simulink model "QD2_IOCheck_AM32ESC_R2022b"  (R2022b)
settings: Solver=ode2  StartTime=0.0  StopTime=inf  FixedStep=1/1000  RelTol=1e-3  EnableMultiTasking=on
undefined symbols (not defined in the file): datetime, HIL, log_QD2_, m, qc_get_step_size, saved_data
libraries: quarc_library x71, simulink x11, simulink_extras x9
(part 2 of 3)

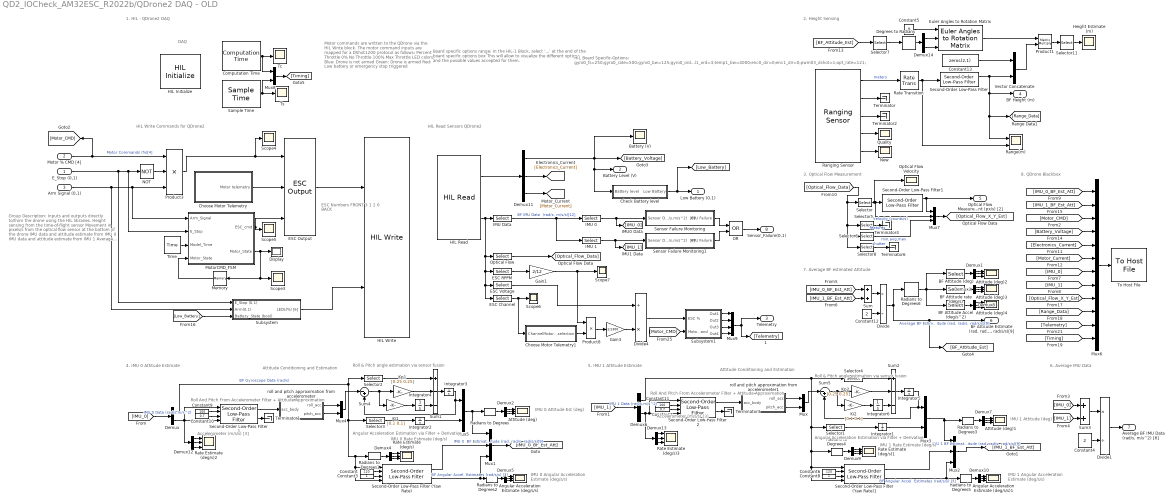
== system QD2_IOCheck_AM32ESC_R2022b/QDrone2 DAQ - OLD ==
  note: 1. HIL - QDrone2 DAQ
  note: HIL Write Commands for QDrone2
  note: ESC Numbers
      |
      | FRONT
      | 3 1
      |
      | 2 0
      | BACK
  note: DAQ
  note: HIL Read Sensors QDrone2
  note: 2. Height Sensing
  note: 3. Optical Flow Measurement
  note: Angular Acceleration Estimation via Filter + Derivative
  note: Roll And Pitch From Accelerometer Filter + Attitude Approximation
  note: Attitude Conditioning and Estimation
  note: 5. IMU 1 Attitude Estimate
  note: IMU 0
      | Rate Estimate (deg/s)
  note: 7. Average BF estimated Attitude
  note: Accelerometer (m/s/s) [3]
  note: Accelerometer (m/s/s) [3]
  note: Roll & Pitch angle estimation via sensor fusion
  note: IMU 1
      | Angular Acceleration
      | Estimate (deg/s/s)
  note: Roll And Pitch From Accelerometer Filter + Attitude Approximation
  note: IMU 1
      | Attitude (deg)
  note: IMU 0
      | Angular Acceleration
      | Estimate (deg/s/s)
  note: Roll & Pitch angle estimation via sensor fusion
  note: Attitude Conditioning and Estimation
  note: 4. IMU 0 Attitude Estimate
  note: IMU 0
      | Attitude Est (deg)
  note: 8. QDrone Blackbox
  note: Angular Acceleration Estimation via Filter + Derivative
  note: 6. Average IMU Data
  note: IMU 1
      | Rate Estimate (deg/s)
  note: Motor commands are written to the QDrone via the HIL Write block. The motor command inputs are mapped for a DShot1200 protocol as follows:
      |
      | Percent Throttle
      | 0% No Throttle
      | 100% Max Throttle
      |
      | LED colors:
      | Blue: Drone is not armed
      | Green: Drone is armed
      | Red: Low battery or emergency stop triggered
  note: Board specific options range:
      |
      | In the HIL-1 Block,
      | select '...' at the end of the board specific options box
      | This will allow to visualize the different options
      | and the possible values accepted for them.
  note: HIL Board Specific-Options:
      | gyro0_fs=250;gyro0_rate=500;gyro0_bw=125;gyro0_ord=3;accel0_fs=16;accel0_rate=1000;accel0_bw=400;accel0_ord=3;temp0_bw=4000;gyro1_fs=250;gyro1_rate=500;gyro1_bw=125;gyro1_ord=3;accel1_fs=16;accel1_rate=1000;accel1_bw=400;accel1_ord=3;temp1_bw=4000;enc0_dir=0;enc1_dir=0;pwm03_dshot=1;opt_rate=121;
  note: Group Description:
      |
      | Inputs and outputs directly to/from the drone using the HIL libraries.
      | Height sensing from the time-of-flight sensor
      | Movement in pixels/s from the optical flow sensor at the bottom of the drone
      | IMU data and attitude estimate from IMU 0
      | IMU data and attitude estimate from IMU 1
      | Average of both IMU outputs
      | Average body frame attitude from IMU data
      | Blackbox saving all relevant values
  E_Stop (0,1) : Inport
  Motor % CMD [4] : Inport  Port=2
  Arm Signal (0,1) : Inport  Port=3
  Angular Acceleration Estimate (deg/s/s) : Scope  NumInputPorts=3
  Angular Acceleration Estimate (deg/s/s)1 : Scope  NumInputPorts=3
  Attitude (deg){,1..4} (5 alike) : Scope  NumInputPorts=3
  BF Attitude (deg) : Selector  InputPortWidth=9  IndexOptions=Index vector (dialog)  Indices=[1:3]  OutputSizes=1
  BF Attitude Accel (deg/s^2) : Selector  InputPortWidth=9  IndexOptions=Index vector (dialog)  Indices=[7:9]  OutputSizes=1
  BF Attitude rate (deg/s) : Selector  InputPortWidth=9  IndexOptions=Index vector (dialog)  Indices=[4:6]  OutputSizes=1
  Battery (V) : Scope
  Check Battery level : Subsystem
  Choose Motor Telemetry : Subsystem
  Choose Motor Telemetry1 : Subsystem
  Computation Time : quarc_library/Sources/Time/Computation Time  sample_time=qc_get_step_size  use_model=on  use_cpu_time=off
  Constant : Constant  Value=120
  Constant10 : Constant  Value=0.7
  Constant11 : Constant  Value=100
  Constant12 : Constant  Value=2
  Constant13 : Constant  Value=zeros(2,1)
  Constant3 : Constant
  Constant4 : Constant  Value=2
  Constant5 : Constant  Value=0
  Constant6 : Constant  Value=120
  Constant7 : Constant  Value=0.7
  Constant8 : Constant
  Constant9 : Constant  Value=100
  Degrees to Radians : simulink_extras/Transformations/Degrees to Radians
  Demux : Demux  Outputs=[3,3]
  Demux{1..5,7..13} (12 alike) : Demux  Outputs=3
  Demux14 : Demux  Outputs=2
  Demux6 : Demux  Outputs=[3,3]
  Display : Display
  Divide : Product  Inputs=*/
  Divide1 : Product  Inputs=*/
  Divide4 : Product  Inputs=/*
  ESC Channel : Selector  InputPortWidth=22  IndexOptions=Index vector (dialog)  Indices=[22]  OutputSizes=1
  ESC Output : quarc_library/Data Acquisition/Generic/Transformations/ESC Output  protocol=DShot (raw)
      settings: AttributesFormatString=%<protocol>  SourceProductName=QUARC Targets
  ESC RPPM : Selector  InputPortWidth=22  IndexOptions=Index vector (dialog)  Indices=[20]  OutputSizes=1
  ESC Voltage : Selector  InputPortWidth=22  IndexOptions=Index vector (dialog)  Indices=[21]  OutputSizes=1
  Euler Angles to Rotation Matrix : quarc_library/Math Operations/Matrices/Euler Angles to Rotation Matrix  menu_order=Relative Z-X-Y
      settings: SourceProductName=QUARC Targets
  Gain1 : Gain  Gain=2/12
  Gain3 : Gain  Gain=1/1300
  HIL Initialize : quarc_library/Data Acquisition/Generic/Configuration/HIL Initialize  object_name=HIL-1  board_type=qdrone2  board_number=0  board_options=gyro0_fs=250;gyro0_rate=500;gyro0_bw=125;gyro0_ord=3;accel0_fs=16;accel0_rate=1000;accel0_bw=400;accel0_ord=3;temp0_bw=4000;gyro1_fs=250;gyro1_rate=500;gyro1_bw=125;gyro1_ord=3;accel1_fs=16;accel1_rate=1000;accel1_bw=400;accel1_ord=3;temp1_bw=4000;enc0_dir=0;enc1_dir=0;pwm03_dshot=1;opt_rate=121;  exclusive=off  active=on  hardware_clocks=[]  clock_modes=[]  initial_clock_frequencies=[]  set_clock_params_at_start=off  set_clock_params_at_switch_in=off  set_clock_frequencies_at_start=off  set_clock_frequencies_at_switch_in=off  analog_input_channels=[0:3]  analog_input_configurations=[]  analog_input_maximums=[3.3]  analog_input_minimums=[0]  set_analog_input_params_at_start=off  set_analog_input_params_at_switch_in=off  analog_output_channels=[]  analog_output_maximums=[]  analog_output_minimums=[]  initial_analog_outputs=[]  final_analog_outputs=[]  watchdog_analog_outputs=[]  set_analog_output_params_at_start=off  set_analog_output_params_at_switch_in=off  set_analog_outputs_at_start=off  set_analog_outputs_at_switch_in=off  set_analog_outputs_at_terminate=off  set_analog_outputs_at_switch_out=off  set_analog_outputs_on_watchdog=off  digital_input_channels=[0:5]  digital_output_channels=[6:11]  digital_output_configuration=[]  initial_digital_outputs=[0]  final_digital_outputs=[0]  watchdog_digital_outputs=[0 0 0 0 0 0]  set_digital_output_params_at_start=off  set_digital_output_params_at_switch_in=off  set_digital_outputs_at_start=on  set_digital_outputs_at_switch_in=off  set_digital_outputs_at_terminate=on  set_digital_outputs_at_switch_out=off  set_digital_outputs_on_watchdog=off  encoder_channels=[0:1]  quadrature=[4]  encoder_filter_frequency=100e6/1  initial_encoder_counts=[0]  set_encoder_params_at_start=on  set_encoder_params_at_switch_in=off  set_encoder_counts_at_start=on  set_encoder_counts_at_switch_in=off  pwm_channels=[0:5]  pwm_modes=[6 6 6 6 0 0]  pwm_frequency=1.2e6  pwm_configuration=[0]  pwm_alignment=[0]  pwm_polarity=[1]  pwm_leading_deadband=[]  pwm_trailing_deadband=[]  initial_pwm_outputs=[0]  final_pwm_outputs=[0]  watchdog_pwm_outputs=[0]  set_pwm_params_at_start=on  set_pwm_params_at_switch_in=off  set_pwm_outputs_at_start=on  set_pwm_outputs_at_switch_in=off  set_pwm_outputs_at_terminate=on  set_pwm_outputs_at_switch_out=off  set_pwm_outputs_on_watchdog=on  other_output_channels=[]  initial_other_outputs=[]  final_other_outputs=[]  watchdog_other_outputs=[]  set_other_outputs_at_start=on  set_other_outputs_at_switch_in=off  set_other_outputs_at_terminate=on  set_other_outputs_at_switch_out=off  set_other_outputs_on_watchdog=off
  HIL Read : quarc_library/Data Acquisition/Generic/Immediate I//O/HIL Read  object_name=HIL-1  analog_channels=[3 1:2]  encoder_channels=[]  digital_channels=[]  other_channels=[3000:3002 4000:4002 3003:3005 4003:4005 17000:17006 17008:17009 17007]  sample_time=qc_get_step_size  active=on  vector_output=on  data_type_mode=Inherit via back propagation  encoder_data_type=double  digital_data_type=boolean
  HIL Write : quarc_library/Data Acquisition/Generic/Immediate I//O/HIL Write  object_name=HIL-1  analog_channels=[]  pwm_channels=[0:3]  digital_channels=[6:11]  other_channels=[]  sample_time=-1  active=off  vector_input=on
  Height Estimate (m) : Scope
  IMU 0 : Selector  InputPortWidth=12  IndexOptions=Index vector (dialog)  Indices=[1:6]  OutputSizes=1
  IMU 1 : Selector  InputPortWidth=12  IndexOptions=Index vector (dialog)  Indices=[7:12]  OutputSizes=1
  IMU Data : Selector  InputPortWidth=22  IndexOptions=Index vector (dialog)  Indices=[1:12]  OutputSizes=1
  Integrator{1..6} (6 alike) : Integrator
  Ki1 : Gain  Gain=[0.1 0.1]
  Ki2 : Gain  Gain=[0.1 0.1]
  Kp1 : Gain  Gain=[0.25 0.25]
  Kp2 : Gain  Gain=[0.25 0.25]
  Memory : Memory
  MotorCMD_FSM : MATLAB Function  TreatAsAtomicUnit=on
  Mux{,3..5,8} (5 alike) : Mux  Inputs=2
  Mux1 : Mux  Inputs=3
  Mux2 : Mux  Inputs=3
  Mux6 : Mux  Inputs=12
  Mux7 : Mux  Inputs=3
  Mux9 : Mux
  NOT : Logic  Operator=NOT  IconShape=distinctive  AllPortsSameDT=off  OutDataTypeStr=boolean
  New : Scope
  OR : Logic  Operator=OR  AllPortsSameDT=off  OutDataTypeStr=boolean
  Optical Flow : Selector  InputPortWidth=22  IndexOptions=Index vector (dialog)  Indices=[13:19]  OutputSizes=1
  Optical Flow Velocity : Scope
  Product1 : Product  Multiplication=Matrix(*)
  Product3 : Product  Inputs=3
  Product8 : Product
  Quality : Scope
  Radians to Degrees{,1..6} (7 alike) : simulink_extras/Transformations/Radians to Degrees
  Range(m) : Scope  NumInputPorts=2
  Ranging Sensor : quarc_library/Devices/Third-Party/Sensors/Ranging Sensor  sensor_type=VL53L1X Time-of-flight  uri=i2c-cpu://localhost:0?address='0x29',baud='400000',memsize='512'  ranging_distance=Long  timing_budget=0.033  measurement_period=0.040  output_mode=Fixed-size output  samples_per_revolution=1300  max_distance=0.050  max_angle=5  sample_time=qc_get_step_size * ceil(1/121/ qc_get_step_size)  show_versions=off  active=on
      settings: SourceProductName=QUARC Targets
  Rate Estimate (deg/s){,1..3} (4 alike) : Scope  NumInputPorts=3
  Rate Transition : RateTransition
  Sample Time : quarc_library/Sources/Time/Sample Time  Priority=-99  sample_time=qc_get_step_size
  Scope{3..7} (5 alike) : Scope
  Second-Order Low-Pass Filter : quarc_library/Continuous/Second-Order Low-Pass Filter  params_source=Internal (dialog parameters)  input_width=100  input_zeta=0.7  input_init=0
  Second-Order Low-Pass Filter (Yaw Rate) : quarc_library/Continuous/Second-Order Low-Pass Filter  params_source=External (input ports)  input_width=200  input_zeta=1  input_init=0
  Second-Order Low-Pass Filter (Yaw Rate)1 : quarc_library/Continuous/Second-Order Low-Pass Filter  params_source=External (input ports)  input_width=200  input_zeta=1  input_init=0
  Second-Order Low-Pass Filter 1 : quarc_library/Continuous/Second-Order Low-Pass Filter  params_source=External (input ports)  input_width=50  input_zeta=1  input_init=0
  Second-Order Low-Pass Filter 2 : quarc_library/Continuous/Second-Order Low-Pass Filter  params_source=External (input ports)  input_width=50  input_zeta=1  input_init=0
  Second-Order Low-Pass Filter1 : quarc_library/Continuous/Second-Order Low-Pass Filter  params_source=Internal (dialog parameters)  input_width=45  input_zeta=1.5  input_init=0
  Selector : Selector  InputPortWidth=7  IndexOptions=Index vector (dialog)  Indices=[1 2]  OutputSizes=1
  Selector1 : Selector  InputPortWidth=3  IndexOptions=Index vector (dialog)  Indices=[3]  OutputSizes=1
  Selector11 : Selector  InputPortWidth=3  IndexOptions=Index vector (dialog)  Indices=[3]  OutputSizes=1
  Selector2 : Selector  InputPortWidth=3  IndexOptions=Index vector (dialog)  Indices=[1,2]  OutputSizes=1
  Selector3 : Selector  InputPortWidth=3  IndexOptions=Index vector (dialog)  Indices=[3]  OutputSizes=1
  Selector4 : Selector  InputPortWidth=3  IndexOptions=Index vector (dialog)  Indices=[1,2]  OutputSizes=1
  Selector5 : Selector  InputPortWidth=7  IndexOptions=Index vector (dialog)  Indices=[3]  OutputSizes=1
  Selector6 : Selector  InputPortWidth=7  IndexOptions=Index vector (dialog)  Indices=[4 5 6]  OutputSizes=1
  Selector7 : Selector  InputPortWidth=9  IndexOptions=Index vector (dialog)  Indices=[1,2]  OutputSizes=1
  Selector8 : Selector  InputPortWidth=7  IndexOptions=Index vector (dialog)  Indices=[7]  OutputSizes=1
  Sensor Failure Monitoring : Subsystem
  Sensor Failure Monitoring1 : Subsystem
  Subsystem : Subsystem
  Subsystem1 : Subsystem
  Sum : Sum
  Sum1 : Sum  Inputs=+--
  Sum2 : Sum  Inputs=+--
  Sum3 : Sum
  Sum4 : Sum  Inputs=|-+
  Sum5 : Sum  Inputs=|-+
  Tc : Scope
  Terminator{,1..4,6} (6 alike) : Terminator
  Time : quarc_library/Sources/Time/Time  time_source=Wall clock  sample_time=qc_get_step_size
  To Host File : quarc_library/Sinks/To Host/To Host File  file_name=saved_data/%m/QDrone2_%{date}_%{time}.mat  variable_name=QDrone_data  decimation=1  sample_time=-1  file_format=MAT-file v.4  options=No header or footer  append=off  final_file_name=saved_data/QDrone2_IO_Check_2021b/QDrone2_10-Apr-2023_14-56-11.mat  bitrate=2000000
  Ts : Scope
  Vector Concatenate : Concatenate
  roll and pitch approximation from accelerometer : MATLAB Function  TreatAsAtomicUnit=on
  roll and pitch approximation from accelerometer1 : MATLAB Function  TreatAsAtomicUnit=on
  Low Battery (0,1) : Outport
  Battery Level (V) : Outport  Port=2
  Telemetry : Outport  Port=3
  "BF Height (m) " : Outport  Port=4
  Optical Flow Measurement (px/s) [2] : Outport  Port=5
  "BF Attitude Estimate (rad, rad/s, rad/s/s)[9]" : Outport  Port=6
  "Average BF IMU Data (rad/s, m/s^2) [6]" : Outport  Port=7
  Sensor_Failure(0,1) : Outport  Port=8
  wires:
  Subsystem/1(LEDs(%) [6]) -> HIL Write/2
  [Low_Battery] -> Subsystem/3(Battery_State (bool))
  Arm Signal (0,1)/1 -> Product3/3, MotorCMD_FSM/1(Arm_Signal), Subsystem/2("Arm(0,1) ")
  NOT/1 -> Product3/2
  Motor % CMD [4]/1 -> [Motor_CMD], Product3/1  "Motor Commands (%)[4]"
  E_Stop (0,1)/1 -> Subsystem/1(E_Stop (0,1)), MotorCMD_FSM/2(E_Stop), NOT/1
  Time/1 -> MotorCMD_FSM/3(Model_Time)
  MotorCMD_FSM/2(Motor_State) -> Scope3/1, Memory/1, Display/1
  Memory/1 -> MotorCMD_FSM/4("Motor_State ")
  Choose Motor Telemetry/1(Motor telemetry) -> ESC Output/2
  ESC Output/1 -> HIL Write/1
  MotorCMD_FSM/1(ESC_cmd) -> ESC Output/3, Scope5/1
  Product3/1 -> Scope4/1, ESC Output/1
  OR/1 -> Sensor_Failure(0,1)/1
  Gain3/1 -> Divide4/2
  [Motor_CMD] -> Subsystem1/2(Motor command)
  ESC Channel/1 -> Scope6/1, Choose Motor Telemetry1/1(Channel)
  HIL Read/2 -> IMU Data/1, ESC RPPM/1, ESC Voltage/1, ESC Channel/1, Optical Flow/1
  ESC RPPM/1 -> Gain1/1
  Gain1/1 -> Product8/1, Scope7/1
  Product8/1 -> Gain3/1
  ESC Voltage/1 -> Divide4/1
  Choose Motor Telemetry1/1(Motor selection) -> Product8/2
  Divide4/1 -> Subsystem1/1(ESC %)
  Check Battery level/1(Low Battery) -> [Low_Battery], Low Battery (0,1)/1
  IMU 1/1 -> [IMU_1], Sensor Failure Monitoring1/1(Sensor Data (rad/s,m/s^2)  [6])
  Sensor Failure Monitoring/1(IMU Failure) -> OR/1
  IMU 0/1 -> [IMU_0], Sensor Failure Monitoring/1(Sensor Data (rad/s,m/s^2)  [6])
  Demux11/1 -> Battery Level (V)/1, Check Battery level/1(Battery level), [Battery_Voltage], Battery (V)/1
  HIL Read/1 -> Demux11/1
  Demux11/3 -> [Motor_Current]
  Demux11/2 -> [Electronics_Current]
  Mux9/1 -> Telemetry/1, [Telemetry]
  Sensor Failure Monitoring1/1(IMU Failure) -> OR/2
  Subsystem1/4(Out4) -> Mux9/4
  IMU Data/1 -> IMU 1/1, IMU 0/1  "BF IMU Data  (rad/s, m/s/s)[12]"
  Subsystem1/2(Out2) -> Mux9/2
  Subsystem1/1(Out1) -> Mux9/1
  Subsystem1/3(Out3) -> Mux9/3
  Optical Flow/1 -> [Optical_Flow_Data]
  Ranging Sensor/2 -> Terminator/1
  Rate Transition/1 -> Range(m)/2, Second-Order Low-Pass Filter/1
  Constant5/1 -> Euler Angles to Rotation Matrix/1
  Selector7/1 -> Degrees to Radians/1
  Euler Angles to Rotation Matrix/1 -> Product1/1
  Ranging Sensor/3 -> Terminator2/1
  Second-Order Low-Pass Filter1/1 -> Optical Flow Measurement (px/s) [2]/1, Mux7/1
  Vector Concatenate/1 -> Product1/2
  Second-Order Low-Pass Filter/1 -> [Range_Data], Range(m)/1, "BF Height (m) "/1, Vector Concatenate/2
  Ranging Sensor/4 -> Quality/1
  Ranging Sensor/1 -> Rate Transition/1  "meters"
  Demux14/2 -> Euler Angles to Rotation Matrix/3
  Product1/1 -> Selector11/1
  Degrees to Radians/1 -> Demux14/1
  Selector11/1 -> Height Estimate (m)/1
  [Optical_Flow_Data] -> Selector/1, Selector8/1, Selector6/1, Selector5/1
  Ranging Sensor/5 -> New/1
  Demux14/1 -> Euler Angles to Rotation Matrix/2
  Constant13/1 -> Vector Concatenate/1
  [BF_Attitude_Est] -> Selector7/1
  BF Attitude rate (deg/s)/1 -> Demux3/1
  Demux12/3 -> Rate Estimate (deg/s)2/3
  Radians to Degrees2/1 -> Demux5/1
  Demux1/1 -> Attitude (deg)2/1
  [IMU_0] -> Sum3/1
  Demux12/1 -> Rate Estimate (deg/s)2/1
  Sum5/1 -> Kp2/1, Ki2/1
  Sum/1 -> Divide/1
  [IMU_1_BF_Est_Att] -> Mux6/2
  [Motor_Current] -> Mux6/6
  [Battery_Voltage] -> Mux6/4
  [IMU_0] -> Mux6/7
  Second-Order Low-Pass Filter (Yaw Rate)1/2 -> Radians to Degrees5/1, Mux2/3  "BF Angular Accel. Estimates (rad/s/s) [3]"
  Sum3/1 -> Divide1/1
  Ki1/1 -> Integrator4/1
  [IMU_0_BF_Est_Att] -> Mux6/1
  Mux6/1 -> To Host File/1
  Integrator4/1 -> Sum1/3
  Integrator3/1 -> Sum4/2, Mux5/1
  Demux7/2 -> Attitude (deg)1/2
  [Electronics_Current] -> Mux6/5
  Demux8/3 -> Attitude (deg)4/3
  Divide1/1 -> "Average BF IMU Data (rad/s, m/s^2) [6]"/1
  Sum4/1 -> Kp1/1, Ki1/1
  Demux3/1 -> Attitude (deg)3/1
  [IMU_0] -> Demux/1  "IMU 0 Data (rad/s,m/s^2)"
  Mux4/1 -> Sum4/1
  Sum2/1 -> Integrator5/1
  [IMU_1_BF_Est_Att] -> Sum/2
  [IMU_0_BF_Est_Att] -> Sum/1
  BF Attitude (deg)/1 -> Demux1/1
  Demux1/2 -> Attitude (deg)2/2
  BF Attitude Accel (deg/s^2)/1 -> Demux8/1
  Demux/1 -> Radians to Degrees1/1, Second-Order Low-Pass Filter (Yaw Rate)/4, Second-Order Low-Pass Filter (Yaw Rate)/1, Selector3/1, Selector2/1  "BF Gyroscope Data (rad/s)"
  Constant11/1 -> Second-Order Low-Pass Filter 2/2
  Constant4/1 -> Divide1/2
  Demux5/2 -> Angular Acceleration Estimate (deg/s/s)/2
  Demux5/1 -> Angular Acceleration Estimate (deg/s/s)/1
  Second-Order Low-Pass Filter 1/1 -> roll and pitch approximation from accelerometer/1(acc_body)
  Demux4/1 -> Rate Estimate (deg/s)/1
  Radians to Degrees5/1 -> Demux10/1
  Demux5/3 -> Angular Acceleration Estimate (deg/s/s)/3
  Integrator6/1 -> Sum2/3
  Demux2/1 -> Attitude (deg)/1
  Selector1/1 -> Integrator1/1
  roll and pitch approximation from accelerometer/1(roll_acc) -> Mux4/1
  Mux/1 -> Sum5/1
  Demux1/3 -> Attitude (deg)2/3
  Sum1/1 -> Integrator3/1
  Selector4/1 -> Sum2/1
  Divide/1 -> Radians to Degrees6/1, [BF_Attitude_Est], "BF Attitude Estimate (rad, rad/s, rad/s/s)[9]"/1  "Average BF Estimated Attitude (rad, rad/s, rad/s/s)[9]"
  Demux2/2 -> Attitude (deg)/2
  roll and pitch approximation from accelerometer1/1(roll_acc) -> Mux/1
  Kp1/1 -> Sum1/2
  Mux3/1 -> Radians to Degrees3/1, Mux2/1
  Radians to Degrees3/1 -> Demux7/1
  Constant/1 -> Second-Order Low-Pass Filter (Yaw Rate)/2
  Demux8/2 -> Attitude (deg)4/2
  Mux5/1 -> Mux1/1, Radians to Degrees/1
  Demux10/1 -> Angular Acceleration Estimate (deg/s/s)1/1
  Mux1/1 -> [IMU_0_BF_Est_Att]  "IMU 0  BF Estimated Attitude (rad, rad/s, rad/s/s)[9]"
  Ki2/1 -> Integrator6/1
  Demux12/2 -> Rate Estimate (deg/s)2/2
  [IMU_1] -> Demux6/1  "IMU 1 Data (rad/s,m/s^2)"
  Demux3/3 -> Attitude (deg)3/3
  Constant6/1 -> Second-Order Low-Pass Filter (Yaw Rate)1/2
  Demux9/3 -> Rate Estimate (deg/s)1/3
  [IMU_1] -> Sum3/2
  roll and pitch approximation from accelerometer1/2(pitch_acc) -> Mux/2
  Demux10/2 -> Angular Acceleration Estimate (deg/s/s)1/2
  Demux/2 -> Demux12/1, Second-Order Low-Pass Filter 1/1, Second-Order Low-Pass Filter 1/4
  Radians to Degrees4/1 -> Demux9/1
  Demux6/1 -> Selector4/1, Second-Order Low-Pass Filter (Yaw Rate)1/4, Second-Order Low-Pass Filter (Yaw Rate)1/1, Radians to Degrees4/1, Selector1/1
  Radians to Degrees1/1 -> Demux4/1
  Integrator5/1 -> Sum5/2, Mux3/1
  Second-Order Low-Pass Filter (Yaw Rate)/2 -> Mux1/3, Radians to Degrees2/1  "BF Angular Accel. Estimates (rad/s/s) [3]"
  Radians to Degrees/1 -> Demux2/1
  Demux4/2 -> Rate Estimate (deg/s)/2
  Demux9/2 -> Rate Estimate (deg/s)1/2
  Selector2/1 -> Sum1/1
  Kp2/1 -> Sum2/2
  Second-Order Low-Pass Filter 2/1 -> roll and pitch approximation from accelerometer1/1(acc_body)
  Second-Order Low-Pass Filter (Yaw Rate)/1 -> Mux1/2
  Constant9/1 -> Second-Order Low-Pass Filter 1/2
  Demux2/3 -> Attitude (deg)/3
  Demux10/3 -> Angular Acceleration Estimate (deg/s/s)1/3
  Demux4/3 -> Rate Estimate (deg/s)/3
  [Range_Data] -> Mux6/10
  Demux3/2 -> Attitude (deg)3/2
  Demux7/3 -> Attitude (deg)1/3
  Integrator2/1 -> Mux5/2
  Constant8/1 -> Second-Order Low-Pass Filter (Yaw Rate)1/3
  roll and pitch approximation from accelerometer/2(pitch_acc) -> Mux4/2
  Constant10/1 -> Second-Order Low-Pass Filter 1/3
  Demux9/1 -> Rate Estimate (deg/s)1/1
  Demux7/1 -> Attitude (deg)1/1
  Integrator1/1 -> Mux3/2
  Second-Order Low-Pass Filter 2/2 -> Terminator3/1
  [Optical_Flow_X_Y_Est] -> Mux6/9
  Constant3/1 -> Second-Order Low-Pass Filter (Yaw Rate)/3
  Constant7/1 -> Second-Order Low-Pass Filter 2/3
  Mux2/1 -> [IMU_1_BF_Est_Att]  "IMU 1 BF Estimated Attitude (rad, rad/s, rad/s/s)[9]"
  Second-Order Low-Pass Filter 1/2 -> Terminator1/1
  Demux8/1 -> Attitude (deg)4/1
  [IMU_1] -> Mux6/8
  Radians to Degrees6/1 -> BF Attitude (deg)/1, BF Attitude rate (deg/s)/1, BF Attitude Accel (deg/s^2)/1
  Selector3/1 -> Integrator2/1
  Constant12/1 -> Divide/2
  Second-Order Low-Pass Filter (Yaw Rate)1/1 -> Mux2/2
  [Motor_CMD] -> Mux6/3
  Sample Time/1 -> Mux8/2, Ts/1
  Computation Time/1 -> Mux8/1, Tc/1
  Selector/1 -> Optical Flow Velocity/1, Mux7/2, Second-Order Low-Pass Filter1/1  "Velocity (counts/s)"
  Demux13/1 -> Rate Estimate (deg/s)3/1
  Demux13/2 -> Rate Estimate (deg/s)3/2
  Demux6/2 -> Demux13/1, Second-Order Low-Pass Filter 2/1, Second-Order Low-Pass Filter 2/4
  Demux13/3 -> Rate Estimate (deg/s)3/3
  Selector5/1 -> Terminator4/1  "features"
  Selector6/1 -> Mux7/3  "min,avg,max"
  Selector8/1 -> Terminator6/1  "shutter"
  Mux7/1 -> [Optical_Flow_X_Y_Est]
  Mux8/1 -> [Timing]
  [Timing] -> Mux6/12
  [Telemetry] -> Mux6/11

== system QD2_IOCheck_AM32ESC_R2022b/QDrone 2 DAQ/Attitude Estimate from IMU Data ==
  IMU Data [12] : Inport
  For Each Subsystem - Iterate over IMU0 and IMU1 : Subsystem  TreatAsAtomicUnit=on
  Reshape into 2 columns for IMU0 and IMU1 : Reshape  OutputDimensionality=Customize  OutputDimensions=[6,2]
  Select Data for IMU0 : Selector  NumberOfDimensions=2  InputPortWidth=3  IndexOptions=Index vector (dialog),Index vector (dialog)  Indices=[1:9],[1]  OutputSizes=1,1
  Select Data for IMU1 : Selector  NumberOfDimensions=2  InputPortWidth=3  IndexOptions=Index vector (dialog),Index vector (dialog)  Indices=[1:9],[2]  OutputSizes=1,1
  "BF Estimated Attitude for IMU0 (rad, rad/s, rad/2^2) [9]" : Outport
  "BF Estimated Attitude for IMU1 (rad, rad/s, rad/2^2) [9]" : Outport  Port=2
  wires:
  IMU Data [12]/1 -> Reshape into 2 columns for IMU0 and IMU1/1
  Reshape into 2 columns for IMU0 and IMU1/1 -> For Each Subsystem - Iterate over IMU0 and IMU1/1(IMU Data [6xn])
  For Each Subsystem - Iterate over IMU0 and IMU1/1("BF Estimated Attitude (rad, rad/s, rad/2^2) [9xn]") -> Select Data for IMU1/1, Select Data for IMU0/1
  Select Data for IMU0/1 -> "BF Estimated Attitude for IMU0 (rad, rad/s, rad/2^2) [9]"/1
  Select Data for IMU1/1 -> "BF Estimated Attitude for IMU1 (rad, rad/s, rad/2^2) [9]"/1

== system QD2_IOCheck_AM32ESC_R2022b/QDrone 2 DAQ/Choose Motor Telemetry ==
  enable telemetry : Inport
  Bias1 : Bias  Bias=0:3  SaturateOnIntegerOverflow=off
  Constant1 : Constant  Value="[0 0 0 0; 1 0 0 0; 0 0 0 0; 0 1 0 0; 0 0 0 0; 0 0 1 0; 0 0 0 0;  0 0 0 1]"
  Constant2 : Constant  Value=8
  Gain : Gain  Gain=.7
  MATLAB Function : MATLAB Function  TreatAsAtomicUnit=on
  Selector : Selector  NumberOfDimensions=2  IndexMode=Zero-based  InputPortWidth=3  IndexOptions=Index vector (port),Select all  Indices=[1 3],1  OutputSizes=1,1
  Telemetry : Scope
  Zero-Order Hold1 : ZeroOrderHold  SampleTime=-1
  Motor telemetry select : Outport
  Motor telemetry index : Outport  Port=2
  wires:
  Gain/1 -> Bias1/1
  Bias1/1 -> Telemetry/1
  MATLAB Function/1(idx) -> Zero-Order Hold1/1
  Zero-Order Hold1/1 -> Selector/2, Motor telemetry index/1
  enable telemetry/1 -> MATLAB Function/1(enable)
  Selector/1 -> Motor telemetry select/1, Gain/1
  Constant1/1 -> Selector/1
  Constant2/1 -> MATLAB Function/2(n)

== system QD2_IOCheck_AM32ESC_R2022b/QDrone 2 DAQ/Construct ESC Speed ==
  ESC Data In [4] : Inport
  ESC Channel Select : Inport  Port=2
  For Each Subsystem - Construct ESC Signal : Subsystem  TreatAsAtomicUnit=on
  Memory : Memory  InitialCondition=zeros(1,4)
  ESC Data Out [4] : Outport
  wires:
  For Each Subsystem - Construct ESC Signal/1(ESC Data Out [4]) -> ESC Data Out [4]/1, Memory/1
  Memory/1 -> For Each Subsystem - Construct ESC Signal/3(ESC Previous Data [4])
  ESC Data In [4]/1 -> For Each Subsystem - Construct ESC Signal/1(ESC Data In [4])
  ESC Channel Select/1 -> For Each Subsystem - Construct ESC Signal/2(ESC Channel)

== system QD2_IOCheck_AM32ESC_R2022b/QDrone 2 DAQ/Construct ESC Temperature ==
  ESC Data In [4] : Inport
  ESC Channel Select : Inport  Port=2
  For Each Subsystem - Construct ESC Signal : Subsystem  TreatAsAtomicUnit=on
  Memory : Memory  InitialCondition=zeros(1,4)
  ESC Data Out [4] : Outport
  wires:
  For Each Subsystem - Construct ESC Signal/1(ESC Data Out [4]) -> ESC Data Out [4]/1, Memory/1
  Memory/1 -> For Each Subsystem - Construct ESC Signal/3(ESC Previous Data [4])
  ESC Data In [4]/1 -> For Each Subsystem - Construct ESC Signal/1(ESC Data In [4])
  ESC Channel Select/1 -> For Each Subsystem - Construct ESC Signal/2(ESC Channel)

== system QD2_IOCheck_AM32ESC_R2022b/QDrone 2 DAQ/Construct ESC Voltage ==
  ESC Data In [4] : Inport
  ESC Channel Select : Inport  Port=2
  For Each Subsystem - Construct ESC Signal : Subsystem  TreatAsAtomicUnit=on
  Memory : Memory  InitialCondition=zeros(1,4)
  ESC Data Out [4] : Outport
  wires:
  ESC Channel Select/1 -> For Each Subsystem - Construct ESC Signal/2(ESC Channel)
  ESC Data In [4]/1 -> For Each Subsystem - Construct ESC Signal/1(ESC Data In [4])
  Memory/1 -> For Each Subsystem - Construct ESC Signal/3(ESC Previous Data [4])
  For Each Subsystem - Construct ESC Signal/1(ESC Data Out [4]) -> Memory/1, ESC Data Out [4]/1

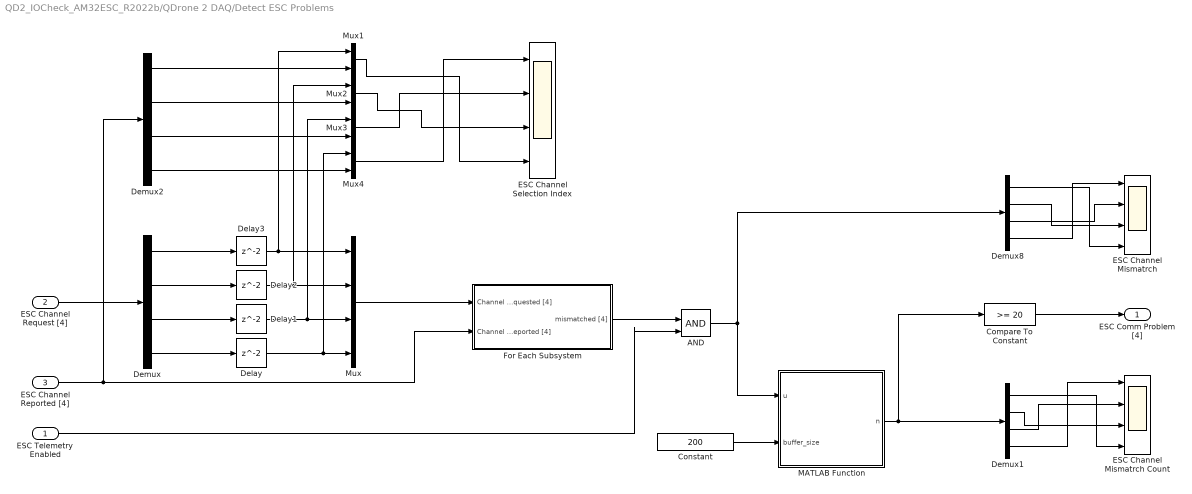
== system QD2_IOCheck_AM32ESC_R2022b/QDrone 2 DAQ/Detect ESC Problems ==
  ESC Telemetry Enabled : Inport
  ESC Channel Request [4] : Inport  Port=2
  ESC Channel Reported [4] : Inport  Port=3
  AND : Logic  IconShape=distinctive  AllPortsSameDT=off  OutDataTypeStr=boolean
  Compare To Constant : simulink/Logic and Bit Operations/Compare To Constant  relop=>=  const=20  OutDataTypeStr=boolean
  Constant : Constant  Value=200
  Delay{,1..3} (4 alike) : Delay
  Demux{,1..2,8} (4 alike) : Demux
  ESC Channel Mismatrch : Scope  NumInputPorts=4
  ESC Channel Mismatrch Count : Scope  NumInputPorts=4
  ESC Channel Selection Index : Scope  NumInputPorts=4
  For Each Subsystem : Subsystem  TreatAsAtomicUnit=on
  MATLAB Function : MATLAB Function  TreatAsAtomicUnit=on
  Mux : Mux
  Mux{1..4} (4 alike) : Mux  Inputs=2
  ESC Comm Problem [4] : Outport
  wires:
  ESC Channel Reported [4]/1 -> Demux2/1, For Each Subsystem/2(Channel Reported [4])
  Demux/1 -> Delay3/1
  Demux/2 -> Delay2/1
  Demux/3 -> Delay1/1
  Demux/4 -> Delay/1
  ESC Channel Request [4]/1 -> Demux/1
  Delay2/1 -> Mux2/1, Mux/2
  Delay3/1 -> Mux/1, Mux1/1
  Delay1/1 -> Mux3/1, Mux/3
  Delay/1 -> Mux4/1, Mux/4
  Mux/1 -> For Each Subsystem/1(Channel Requested [4])
  For Each Subsystem/1(mismatched [4]) -> AND/1
  AND/1 -> MATLAB Function/1(u), Demux8/1
  Demux8/2 -> ESC Channel Mismatrch/3
  Demux8/1 -> ESC Channel Mismatrch/4
  Demux8/3 -> ESC Channel Mismatrch/2
  Demux8/4 -> ESC Channel Mismatrch/1
  Constant/1 -> MATLAB Function/2(buffer_size)
  Demux1/4 -> ESC Channel Mismatrch Count/1
  Demux1/3 -> ESC Channel Mismatrch Count/2
  Demux1/1 -> ESC Channel Mismatrch Count/4
  Demux1/2 -> ESC Channel Mismatrch Count/3
  MATLAB Function/1(n) -> Compare To Constant/1, Demux1/1
  Compare To Constant/1 -> ESC Comm Problem [4]/1
  ESC Telemetry Enabled/1 -> AND/2
  Demux2/1 -> Mux1/2
  Demux2/2 -> Mux2/2
  Demux2/3 -> Mux3/2
  Demux2/4 -> Mux4/2
  Mux4/1 -> ESC Channel Selection Index/1
  Mux3/1 -> ESC Channel Selection Index/2
  Mux2/1 -> ESC Channel Selection Index/3
  Mux1/1 -> ESC Channel Selection Index/4

== system QD2_IOCheck_AM32ESC_R2022b/QDrone 2 DAQ/Enabled Subsystem - Write ESC Commands ==
  DShot Raw [4] : Inport
  Enable : EnablePort
  HIL Write PWM : quarc_library/Data Acquisition/Generic/Immediate I//O/HIL Write PWM  object_name=HIL-1  channels=[0:3]  sample_time=-1  active=off  vector_input=on
      settings: AttributesFormatString=(%<object_name>)  SourceProductName=QUARC Targets
  wires:
  DShot Raw [4]/1 -> HIL Write PWM/1

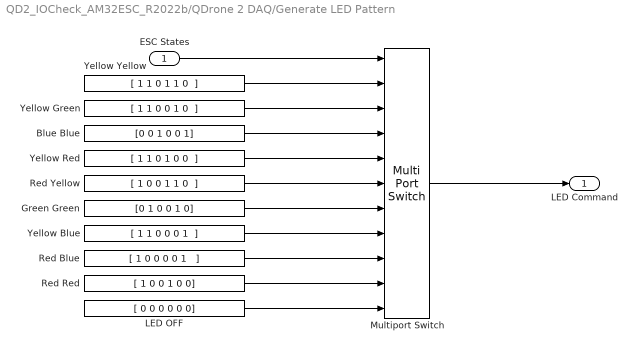
== system QD2_IOCheck_AM32ESC_R2022b/QDrone 2 DAQ/Generate LED Pattern ==
  ESC States : Inport
  Blue Blue : Constant  Value=[0 0 1 0 0 1]
  Green Green : Constant  Value=[0 1 0 0 1 0]
  LED OFF : Constant  Value=[ 0 0 0 0 0 0]
  Multiport Switch : MultiPortSwitch  DataPortOrder=Specify indices  DataPortIndices={0,1,2,3,4,5,77,88,99}  DataPortForDefault=Additional data port  DiagnosticForDefault=Warning  SaturateOnIntegerOverflow=off  InputSameDT=off
  Red Blue : Constant  Value="[ 1 0 0 0 0 1   ]"
  Red Red : Constant  Value=[ 1 0 0 1 0 0]
  Red Yellow : Constant  Value="[ 1 0 0 1 1 0  ]"
  Yellow Blue : Constant  Value="[ 1 1 0 0 0 1  ]"
  Yellow Green : Constant  Value="[ 1 1 0 0 1 0  ]"
  Yellow Red : Constant  Value="[ 1 1 0 1 0 0  ]"
  Yellow Yellow : Constant  Value="[ 1 1 0 1 1 0  ]"
  LED Command : Outport
  wires:
  Multiport Switch/1 -> LED Command/1
  ESC States/1 -> Multiport Switch/1
  Blue Blue/1 -> Multiport Switch/4
  Red Red/1 -> Multiport Switch/10
  Yellow Yellow/1 -> Multiport Switch/2
  Red Blue/1 -> Multiport Switch/9
  Yellow Blue/1 -> Multiport Switch/8
  LED OFF/1 -> Multiport Switch/11
  Green Green/1 -> Multiport Switch/7
  Yellow Green/1 -> Multiport Switch/3
  Yellow Red/1 -> Multiport Switch/5
  Red Yellow/1 -> Multiport Switch/6

== system QD2_IOCheck_AM32ESC_R2022b/QDrone 2 DAQ/Monitor Battery Level ==
  note: Monitor Battery Level.
      | Flag Low Battery Error if
      | Battery level dips below
      | threshold for specified
      | threshold time period.
  Battery (V) : Inport
  AND : Logic  IconShape=distinctive  AllPortsSameDT=off  OutDataTypeStr=boolean
  Battery Low Time Threshold (s) : Constant  Value=0.3
  Constant : Constant  Value=0.5
  Data Type Conversion : DataTypeConversion  SaturateOnIntegerOverflow=off  RndMeth=Floor
  Data Type Conversion1 : DataTypeConversion  SaturateOnIntegerOverflow=off  RndMeth=Floor
  Greater than minimum expected voltage (Valid Battery Reading) : simulink/Logic and Bit Operations/Compare To Constant  relop=>  const=0.5  OutDataTypeStr=boolean
  Less than minimum threshold voltage (Battery level too low) : simulink/Logic and Bit Operations/Compare To Constant  relop=<=  const=14  OutDataTypeStr=boolean
  Terminator : Terminator
  Threshold : quarc_library/Discontinuities/Threshold  operator=>=  param_src=External input port  threshold=0  duration=0
      settings: SourceProductName=QUARC Targets
  Triggered Subsystem - Latching Flag : Subsystem  TreatAsAtomicUnit=on
  Low Battery : Outport
  wires:
  Battery (V)/1 -> Less than minimum threshold voltage (Battery level too low)/1, Greater than minimum expected voltage (Valid Battery Reading)/1
  Less than minimum threshold voltage (Battery level too low)/1 -> AND/2
  Greater than minimum expected voltage (Valid Battery Reading)/1 -> AND/1
  AND/1 -> Data Type Conversion/1
  Constant/1 -> Threshold/2
  Battery Low Time Threshold (s)/1 -> Threshold/3
  Data Type Conversion/1 -> Threshold/1
  Threshold/2 -> Terminator/1
  Threshold/1 -> Triggered Subsystem - Latching Flag/Trigger
  Triggered Subsystem - Latching Flag/1(Out1) -> Data Type Conversion1/1
  Data Type Conversion1/1 -> Low Battery/1

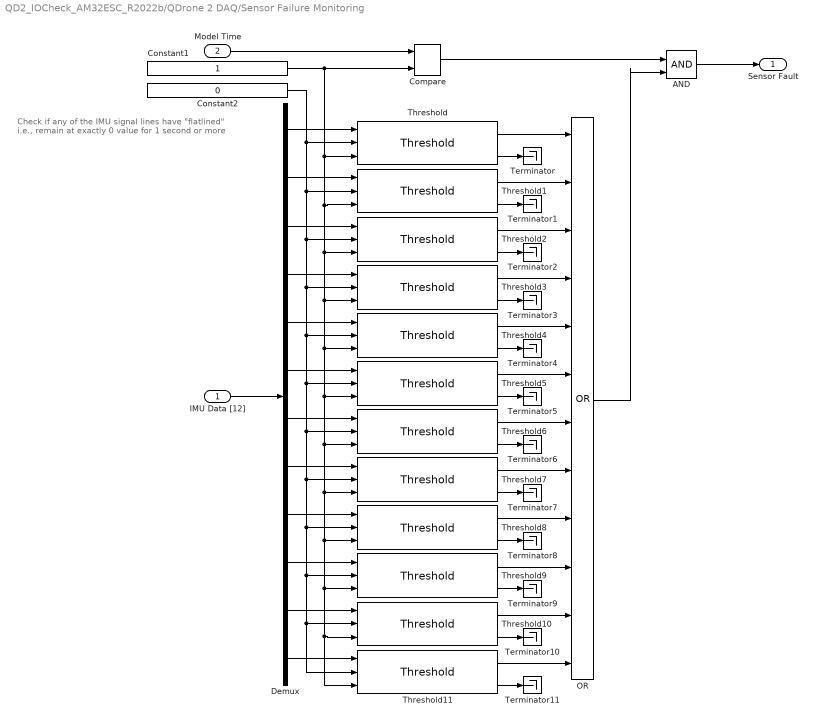
== system QD2_IOCheck_AM32ESC_R2022b/QDrone 2 DAQ/Sensor Failure Monitoring ==
  note: Check if any of the IMU signal lines have "flatlined"
      | i.e., remain at exactly 0 value for 1 second or more
  IMU Data [12] : Inport
  Model Time : Inport  Port=2
  AND : Logic  IconShape=distinctive  AllPortsSameDT=off  OutDataTypeStr=boolean
  Compare : quarc_library/Logic Operations/Compare  operator=>=  output_data_type=boolean
      settings: SourceProductName=QUARC Targets
  Constant1 : Constant
  Constant2 : Constant  Value=0
  Demux : Demux  Outputs=12
  OR : Logic  Operator=OR  Inputs=12  AllPortsSameDT=off  OutDataTypeStr=boolean
  Terminator{,1..11} (12 alike) : Terminator
  Threshold{,1..11} (12 alike) : quarc_library/Discontinuities/Threshold  operator===  param_src=External input port  threshold=0  duration=1
      settings: SourceProductName=QUARC Targets
  Sensor Fault : Outport
  wires:
  Model Time/1 -> Compare/1
  Constant1/1 -> Threshold1/3, Threshold2/3, Threshold3/3, Threshold5/3, Threshold6/3, Threshold7/3, Threshold8/3, Threshold9/3, Threshold10/3, Threshold11/3, Threshold4/3, Threshold/3, Compare/2
  Demux/1 -> Threshold/1
  Demux/2 -> Threshold1/1
  Constant2/1 -> Threshold1/2, Threshold2/2, Threshold3/2, Threshold4/2, Threshold5/2, Threshold6/2, Threshold7/2, Threshold8/2, Threshold9/2, Threshold10/2, Threshold11/2, Threshold/2
  IMU Data [12]/1 -> Demux/1
  Demux/3 -> Threshold2/1
  Demux/4 -> Threshold3/1
  Demux/5 -> Threshold4/1
  Demux/6 -> Threshold5/1
  Demux/7 -> Threshold6/1
  Demux/8 -> Threshold7/1
  Demux/9 -> Threshold8/1
  Demux/10 -> Threshold9/1
  Demux/11 -> Threshold10/1
  Demux/12 -> Threshold11/1
  Threshold/1 -> OR/1
  Threshold1/1 -> OR/2
  Threshold2/1 -> OR/3
  Threshold3/1 -> OR/4
  Threshold4/1 -> OR/5
  Threshold5/1 -> OR/6
  Threshold6/1 -> OR/7
  Threshold7/1 -> OR/8
  Threshold8/1 -> OR/9
  Threshold9/1 -> OR/10
  Threshold10/1 -> OR/11
  Threshold11/1 -> OR/12
  Threshold/2 -> Terminator/1
  Threshold1/2 -> Terminator1/1
  Threshold2/2 -> Terminator2/1
  Threshold3/2 -> Terminator3/1
  Threshold4/2 -> Terminator4/1
  Threshold5/2 -> Terminator5/1
  Threshold6/2 -> Terminator6/1
  Threshold7/2 -> Terminator7/1
  Threshold8/2 -> Terminator8/1
  Threshold9/2 -> Terminator9/1
  Threshold10/2 -> Terminator10/1
  Threshold11/2 -> Terminator11/1
  Compare/1 -> AND/1
  OR/1 -> AND/2
  AND/1 -> Sensor Fault/1

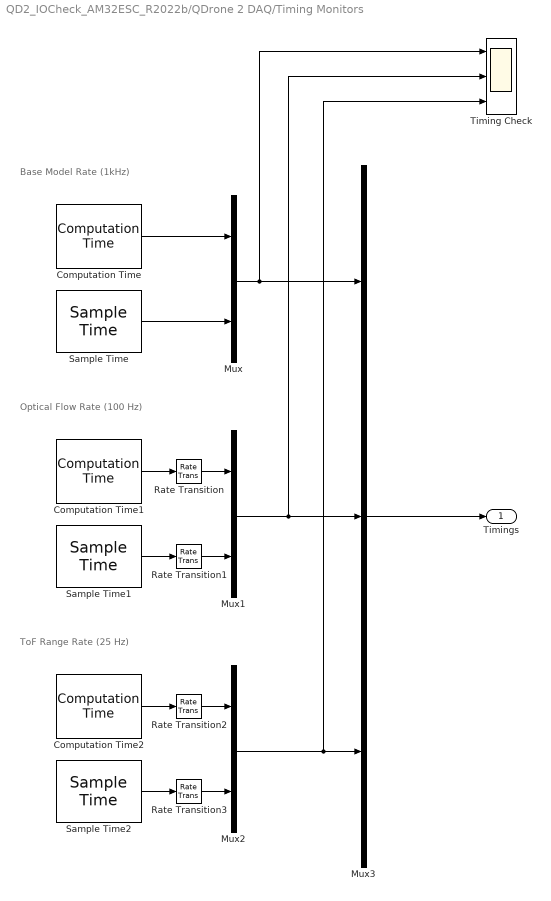
== system QD2_IOCheck_AM32ESC_R2022b/QDrone 2 DAQ/Timing Monitors ==
  note: Base Model Rate (1kHz)
  note: Optical Flow Rate (100 Hz)
  note: ToF Range Rate (25 Hz)
  Computation Time : quarc_library/Sources/Time/Computation Time  sample_time=qc_get_step_size  use_model=on  use_cpu_time=off
  Computation Time1 : quarc_library/Sources/Time/Computation Time  sample_time=0.01  use_model=on  use_cpu_time=off
  Computation Time2 : quarc_library/Sources/Time/Computation Time  sample_time=0.04  use_model=on  use_cpu_time=off
  Mux : Mux  Inputs=2
  Mux1 : Mux  Inputs=2
  Mux2 : Mux  Inputs=2
  Mux3 : Mux  Inputs=3
  Rate Transition{,1..3} (4 alike) : RateTransition
  Sample Time : quarc_library/Sources/Time/Sample Time  Priority=-99  sample_time=qc_get_step_size
  Sample Time1 : quarc_library/Sources/Time/Sample Time  Priority=-99  sample_time=0.01
  Sample Time2 : quarc_library/Sources/Time/Sample Time  Priority=-99  sample_time=0.04
  Timing Check : Scope  NumInputPorts=3
  Timings : Outport
  wires:
  Computation Time/1 -> Mux/1
  Sample Time/1 -> Mux/2
  Sample Time1/1 -> Rate Transition1/1
  Computation Time1/1 -> Rate Transition/1
  Computation Time2/1 -> Rate Transition2/1
  Sample Time2/1 -> Rate Transition3/1
  Mux1/1 -> Mux3/2, Timing Check/2
  Mux/1 -> Timing Check/1, Mux3/1
  Mux2/1 -> Timing Check/3, Mux3/3
  Mux3/1 -> Timings/1
  Rate Transition/1 -> Mux1/1
  Rate Transition1/1 -> Mux1/2
  Rate Transition2/1 -> Mux2/1
  Rate Transition3/1 -> Mux2/2

== system QD2_IOCheck_AM32ESC_R2022b/QDrone2 DAQ - OLD/Check Battery level ==
  Battery level : Inport
  Compare To Constant : simulink/Logic and Bit Operations/Compare To Constant  relop=<=  const=14  OutDataTypeStr=boolean
  Compare To Constant1 : simulink/Logic and Bit Operations/Compare To Constant  relop=>  const=0.5  OutDataTypeStr=boolean
  Data Type Conversion : DataTypeConversion  SaturateOnIntegerOverflow=off  RndMeth=Floor
  Data Type Conversion1 : DataTypeConversion  SaturateOnIntegerOverflow=off  RndMeth=Floor
  Logical Operator : Logic  AllPortsSameDT=off  OutDataTypeStr=boolean
  Terminator : Terminator
  Threshold : quarc_library/Discontinuities/Threshold  operator=>=  param_src=Specify via dialog  threshold=0.5  duration=0.3
      settings: SourceProductName=QUARC Targets
  Triggered Subsystem : Subsystem  TreatAsAtomicUnit=on
  Low Battery : Outport  VectorParamsAs1DForOutWhenUnconnected=off
  wires:
  Threshold/2 -> Terminator/1
  Battery level/1 -> Compare To Constant1/1, Compare To Constant/1
  Threshold/1 -> Logical Operator/2
  Logical Operator/1 -> Triggered Subsystem/Trigger
  Compare To Constant1/1 -> Logical Operator/1
  Compare To Constant/1 -> Data Type Conversion/1
  Data Type Conversion/1 -> Threshold/1
  Data Type Conversion1/1 -> Low Battery/1
  Triggered Subsystem/1(Out1) -> Data Type Conversion1/1

== system QD2_IOCheck_AM32ESC_R2022b/QDrone2 DAQ - OLD/Choose Motor Telemetry ==
  Bias1 : Bias  Bias=0:3  SaturateOnIntegerOverflow=off
  Constant : Constant  Value=[0 0 0 0; 0 0 0 1; 0 0 0 0; 0 0 1 0; 0 0 0 0; 0 1 0 0; 0 0 0 0; 1 0 0 0]
  Counter Free-Running : simulink/Sources/Counter Free-Running  NumBits=3  tsamp=-1
  Gain : Gain  Gain=.7
  Selector : Selector  NumberOfDimensions=2  IndexMode=Zero-based  InputPortWidth=3  IndexOptions=Index vector (port),Select all  Indices=[1 3],1  OutputSizes=1,1
  Telemetry : Scope
  Motor telemetry : Outport
  wires:
  Gain/1 -> Bias1/1
  Bias1/1 -> Telemetry/1
  Constant/1 -> Selector/1
  Counter Free-Running/1 -> Selector/2
  Selector/1 -> Motor telemetry/1, Gain/1

== system QD2_IOCheck_AM32ESC_R2022b/QDrone2 DAQ - OLD/Choose Motor Telemetry1 ==
  Channel : Inport
  Constant1 : Constant  Value=[1 0 0 0]
  Constant2 : Constant  Value=[0 1 0 0]
  Constant3 : Constant  Value=[0 0 1 0]
  Constant4 : Constant  Value=[0 0 0 1]
  Multiport Switch : MultiPortSwitch  DataPortOrder=Zero-based contiguous  Inputs=4  zeroidx=on  SaturateOnIntegerOverflow=off  InputSameDT=off
  Motor selection : Outport
  wires:
  Multiport Switch/1 -> Motor selection/1
  Constant4/1 -> Multiport Switch/5
  Constant3/1 -> Multiport Switch/4
  Constant1/1 -> Multiport Switch/2
  Constant2/1 -> Multiport Switch/3
  Channel/1 -> Multiport Switch/1

== system QD2_IOCheck_AM32ESC_R2022b/QDrone2 DAQ - OLD/Sensor Failure Monitoring ==
  note: Check for no data condition (flat-line zero) from any of the onboard sensors
  Sensor Data (rad/s,m/s^2)  [6] : Inport
  Data Type Conversion1 : DataTypeConversion  SaturateOnIntegerOverflow=off  RndMeth=Floor
  Data Type Conversion2 : DataTypeConversion  SaturateOnIntegerOverflow=off  RndMeth=Floor
  Data Type Conversion4 : DataTypeConversion  SaturateOnIntegerOverflow=off  RndMeth=Floor
  Demux : Demux  Outputs=[3 3]
  Logical Operator : Logic  Operator=OR  Inputs=1  AllPortsSameDT=off  OutDataTypeStr=boolean
  Mux : Mux  Inputs=2
  Sensor Failure (Accelerometer) : Subsystem
  Sensor Failure (Gyroscope) : Subsystem
  IMU Failure : Outport  VectorParamsAs1DForOutWhenUnconnected=off
  wires:
  Data Type Conversion4/1 -> IMU Failure/1
  Logical Operator/1 -> Data Type Conversion4/1
  Demux/1 -> Sensor Failure (Gyroscope)/1(Sensor Input)
  Data Type Conversion1/1 -> Mux/2
  Data Type Conversion2/1 -> Mux/1
  Mux/1 -> Logical Operator/1
  Sensor Failure (Accelerometer)/1(Sensor Fault) -> Data Type Conversion1/1
  Sensor Failure (Gyroscope)/1(Sensor Fault) -> Data Type Conversion2/1
  Demux/2 -> Sensor Failure (Accelerometer)/1(Sensor Input)
  Sensor Data (rad/s,m/s^2)  [6]/1 -> Demux/1

== system QD2_IOCheck_AM32ESC_R2022b/QDrone2 DAQ - OLD/Sensor Failure Monitoring1 ==
  note: Check for no data condition (flat-line zero) from any of the onboard sensors
  Sensor Data (rad/s,m/s^2)  [6] : Inport
  Data Type Conversion1 : DataTypeConversion  SaturateOnIntegerOverflow=off  RndMeth=Floor
  Data Type Conversion2 : DataTypeConversion  SaturateOnIntegerOverflow=off  RndMeth=Floor
  Data Type Conversion4 : DataTypeConversion  SaturateOnIntegerOverflow=off  RndMeth=Floor
  Demux : Demux  Outputs=[3 3]
  Logical Operator : Logic  Operator=OR  Inputs=1  AllPortsSameDT=off  OutDataTypeStr=boolean
  Mux : Mux  Inputs=2
  Sensor Failure (Accelerometer) : Subsystem
  Sensor Failure (Gyroscope) : Subsystem
  IMU Failure : Outport  VectorParamsAs1DForOutWhenUnconnected=off
  wires:
  Sensor Data (rad/s,m/s^2)  [6]/1 -> Demux/1
  Demux/2 -> Sensor Failure (Accelerometer)/1(Sensor Input)
  Sensor Failure (Gyroscope)/1(Sensor Fault) -> Data Type Conversion2/1
  Sensor Failure (Accelerometer)/1(Sensor Fault) -> Data Type Conversion1/1
  Mux/1 -> Logical Operator/1
  Data Type Conversion2/1 -> Mux/1
  Data Type Conversion1/1 -> Mux/2
  Demux/1 -> Sensor Failure (Gyroscope)/1(Sensor Input)
  Logical Operator/1 -> Data Type Conversion4/1
  Data Type Conversion4/1 -> IMU Failure/1

== system QD2_IOCheck_AM32ESC_R2022b/QDrone2 DAQ - OLD/Subsystem ==
  note: PCB LED 2
  note: PCB LED 1
  E_Stop (0,1) : Inport
  "Arm(0,1) " : Inport  Port=2
  Battery_State (bool) : Inport  Port=3
  Blue : Constant  Value=[0 0 1]
  Green : Constant  Value=[0 1 0]
  MATLAB Function LED Color Assignment : MATLAB Function  TreatAsAtomicUnit=on
  Multiport Switch : MultiPortSwitch  SaturateOnIntegerOverflow=off  InputSameDT=off
  Mux : Mux  Inputs=2
  Red : Constant  Value=[1 0 0]
  LEDs(%) [6] : Outport
  wires:
  Mux/1 -> LEDs(%) [6]/1
  Multiport Switch/1 -> Mux/1, Mux/2
  Blue/1 -> Multiport Switch/4
  Green/1 -> Multiport Switch/3
  Red/1 -> Multiport Switch/2
  Battery_State (bool)/1 -> MATLAB Function LED Color Assignment/3(low_battery)
  E_Stop (0,1)/1 -> MATLAB Function LED Color Assignment/1(E_Stop)
  "Arm(0,1) "/1 -> MATLAB Function LED Color Assignment/2(Arm)
  MATLAB Function LED Color Assignment/1(value) -> Multiport Switch/1

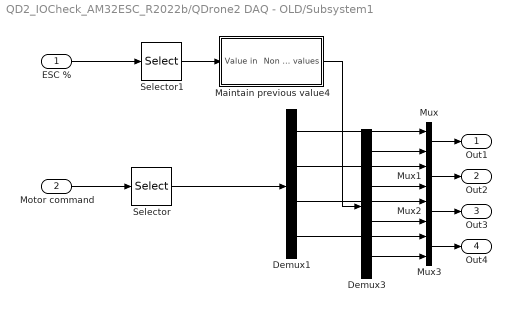
== system QD2_IOCheck_AM32ESC_R2022b/QDrone2 DAQ - OLD/Subsystem1 ==
  ESC % : Inport
  Motor command : Inport  Port=2
  Demux1 : Demux
  Demux3 : Demux
  Maintain previous value4 : Subsystem
  Mux{,1..3} (4 alike) : Mux  Inputs=2
  Selector : Selector  InputPortWidth=4  IndexOptions=Index vector (dialog)  Indices=[4 3 2 1]  OutputSizes=1
  Selector1 : Selector  InputPortWidth=4  IndexOptions=Index vector (dialog)  Indices=[4 3 2 1]  OutputSizes=1
  Out1 : Outport
  Out2 : Outport  Port=2
  Out3 : Outport  Port=3
  Out4 : Outport  Port=4
  wires:
  Motor command/1 -> Selector/1
  Demux1/2 -> Mux1/1
  Selector/1 -> Demux1/1
  Demux1/1 -> Mux/1
  Demux1/4 -> Mux3/1
  Demux1/3 -> Mux2/1
  Mux3/1 -> Out4/1
  Mux2/1 -> Out3/1
  Mux/1 -> Out1/1
  Mux1/1 -> Out2/1
  ESC %/1 -> Selector1/1
  Demux3/1 -> Mux/2
  Demux3/2 -> Mux1/2
  Demux3/3 -> Mux2/2
  Demux3/4 -> Mux3/2
  Selector1/1 -> Maintain previous value4/1(Value in)
  Maintain previous value4/1(Non 0 values) -> Demux3/1

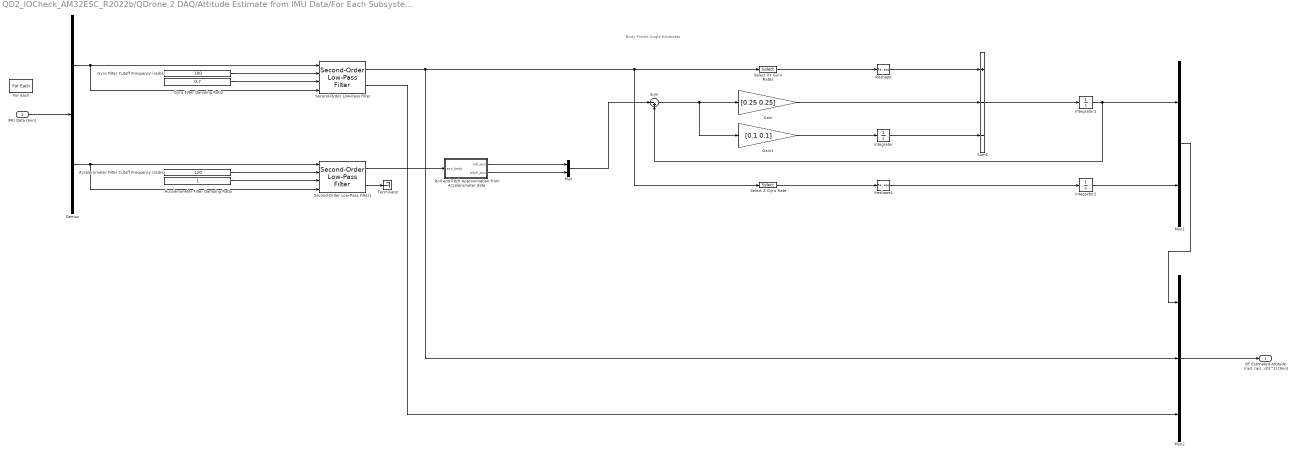
== system QD2_IOCheck_AM32ESC_R2022b/QDrone 2 DAQ/Attitude Estimate from IMU Data/For Each Subsystem - Iterate over IMU0 and IMU1 ==
  note: Body Frame Angle Estimates
  IMU Data [6xn] : Inport  Partition=on  PartitionDimension=2  PartitionWidth=1  PartitionOffset=0
  Accelerometer Filter Cutoff Frequency (rad/s) : Constant  Value=120
  Accelerometer Filter Damping Ratio : Constant
  Demux : Demux  Outputs=[3, 3]
  For Each : ForEach  DisableCoverage=on
  Gain : Gain  Gain=[0.25 0.25]
  Gain1 : Gain  Gain=[0.1 0.1]
  Gyro Filter Cutoff Frequency (rad/s) : Constant  Value=100
  Gyro Filter Damping Ratio : Constant  Value=0.7
  Integrator : Integrator
  Integrator1 : Integrator
  Integrator2 : Integrator
  Mux : Mux  Inputs=2
  Mux1 : Mux  Inputs=2
  Mux2 : Mux  Inputs=3
  Reshape : Reshape
  Reshape1 : Reshape
  Roll and Pitch Approximation from Accelerometer data : MATLAB Function  TreatAsAtomicUnit=on
  Second-Order Low-Pass Filter : quarc_library/Continuous/Second-Order Low-Pass Filter  params_source=External (input ports)  input_width=1  input_zeta=1  input_init=0
  Second-Order Low-Pass Filter1 : quarc_library/Continuous/Second-Order Low-Pass Filter  params_source=External (input ports)  input_width=1  input_zeta=1  input_init=0
  Select XY Gyro Rates : Selector  InputPortWidth=3  IndexOptions=Index vector (dialog)  Indices=[1 2]  OutputSizes=1
  Select Z Gyro Rate : Selector  InputPortWidth=3  IndexOptions=Index vector (dialog)  Indices=[3]  OutputSizes=1
  Sum : Sum  Inputs=|-+
  Sum1 : Sum  Inputs=+--
  Terminator : Terminator
  "BF Estimated Attitude (rad, rad/s, rad/2^2) [9xn]" : Outport  ConcatenationDimension=2
  wires:
  IMU Data [6xn]/1 -> Demux/1
  Demux/1 -> Second-Order Low-Pass Filter/4, Second-Order Low-Pass Filter/1
  Gyro Filter Cutoff Frequency (rad/s)/1 -> Second-Order Low-Pass Filter/2
  Gyro Filter Damping Ratio/1 -> Second-Order Low-Pass Filter/3
  Accelerometer Filter Damping Ratio/1 -> Second-Order Low-Pass Filter1/3
  Accelerometer Filter Cutoff Frequency (rad/s)/1 -> Second-Order Low-Pass Filter1/2
  Demux/2 -> Second-Order Low-Pass Filter1/4, Second-Order Low-Pass Filter1/1
  Second-Order Low-Pass Filter1/1 -> Roll and Pitch Approximation from Accelerometer data/1(acc_body)
  Second-Order Low-Pass Filter1/2 -> Terminator/1
  Roll and Pitch Approximation from Accelerometer data/1(roll_acc) -> Mux/1
  Roll and Pitch Approximation from Accelerometer data/2(pitch_acc) -> Mux/2
  Mux/1 -> Sum/1
  Sum/1 -> Gain1/1, Gain/1
  Gain1/1 -> Integrator/1
  Integrator/1 -> Sum1/3
  Gain/1 -> Sum1/2
  Second-Order Low-Pass Filter/1 -> Mux2/2, Select Z Gyro Rate/1, Select XY Gyro Rates/1
  Select XY Gyro Rates/1 -> Reshape/1
  Sum1/1 -> Integrator1/1
  Integrator1/1 -> Mux1/1, Sum/2
  Select Z Gyro Rate/1 -> Reshape1/1
  Integrator2/1 -> Mux1/2
  Mux1/1 -> Mux2/1
  Mux2/1 -> "BF Estimated Attitude (rad, rad/s, rad/2^2) [9xn]"/1
  Second-Order Low-Pass Filter/2 -> Mux2/3
  Reshape/1 -> Sum1/1
  Reshape1/1 -> Integrator2/1

== system QD2_IOCheck_AM32ESC_R2022b/QDrone 2 DAQ/Construct ESC Speed/For Each Subsystem - Construct ESC Signal ==
  ESC Data In [4] : Inport  Partition=on  PartitionDimension=1  PartitionWidth=1  PartitionOffset=0
  ESC Channel : Inport  Port=2
  ESC Previous Data [4] : Inport  Port=3  Partition=on  PartitionDimension=1  PartitionWidth=1  PartitionOffset=0
  Compare : quarc_library/Logic Operations/Compare  operator===  output_data_type=boolean
      settings: SourceProductName=QUARC Targets
  For Each : ForEach  DisableCoverage=on  ShowIterationIndex=on
  Switch : Switch  Criteria=u2 ~= 0  SaturateOnIntegerOverflow=off  InputSameDT=off
  ESC Data Out [4] : Outport  ConcatenationDimension=1
  wires:
  ESC Data In [4]/1 -> Switch/1
  Switch/1 -> ESC Data Out [4]/1
  ESC Channel/1 -> Compare/2
  For Each/1 -> Compare/1
  Compare/1 -> Switch/2
  ESC Previous Data [4]/1 -> Switch/3

== system QD2_IOCheck_AM32ESC_R2022b/QDrone 2 DAQ/Construct ESC Temperature/For Each Subsystem - Construct ESC Signal ==
  ESC Data In [4] : Inport  Partition=on  PartitionDimension=1  PartitionWidth=1  PartitionOffset=0
  ESC Channel : Inport  Port=2
  ESC Previous Data [4] : Inport  Port=3  Partition=on  PartitionDimension=1  PartitionWidth=1  PartitionOffset=0
  Compare : quarc_library/Logic Operations/Compare  operator===  output_data_type=boolean
      settings: SourceProductName=QUARC Targets
  For Each : ForEach  DisableCoverage=on  ShowIterationIndex=on
  Switch : Switch  Criteria=u2 ~= 0  SaturateOnIntegerOverflow=off  InputSameDT=off
  ESC Data Out [4] : Outport  ConcatenationDimension=1
  wires:
  ESC Data In [4]/1 -> Switch/1
  Switch/1 -> ESC Data Out [4]/1
  ESC Channel/1 -> Compare/2
  For Each/1 -> Compare/1
  Compare/1 -> Switch/2
  ESC Previous Data [4]/1 -> Switch/3

== system QD2_IOCheck_AM32ESC_R2022b/QDrone 2 DAQ/Construct ESC Voltage/For Each Subsystem - Construct ESC Signal ==
  ESC Data In [4] : Inport  Partition=on  PartitionDimension=1  PartitionWidth=1  PartitionOffset=0
  ESC Channel : Inport  Port=2
  ESC Previous Data [4] : Inport  Port=3  Partition=on  PartitionDimension=1  PartitionWidth=1  PartitionOffset=0
  Compare : quarc_library/Logic Operations/Compare  operator===  output_data_type=boolean
      settings: SourceProductName=QUARC Targets
  For Each : ForEach  DisableCoverage=on  ShowIterationIndex=on
  Switch : Switch  Criteria=u2 ~= 0  SaturateOnIntegerOverflow=off  InputSameDT=off
  ESC Data Out [4] : Outport  ConcatenationDimension=1
  wires:
  ESC Previous Data [4]/1 -> Switch/3
  Compare/1 -> Switch/2
  For Each/1 -> Compare/1
  ESC Channel/1 -> Compare/2
  Switch/1 -> ESC Data Out [4]/1
  ESC Data In [4]/1 -> Switch/1
